simulink model "gm_combinedTxRx_ExternalMode"  (R2017b)
settings: Solver=FixedStepDiscrete  StartTime=0.0  StopTime=10.0  RelTol=1e-3
InitFcn:
  | modelSettings
undefined symbols (not defined in the file or in its folder): coeff, filt, j, RadioSampleRate, VibertiTracebackLength, xPreambleSeq
libraries: simulink x20, dsphdlfiltering x20, hdlsllib x10, hdlmdlgenlib x6, dspsigops x5, commseqgen3 x4, commdigbbndpm3 x3, commcrc2 x2, commcnvcod2 x2, commsource2 x1, dspstat3 x1, dspmlti4 x1
(part 4 of 5)

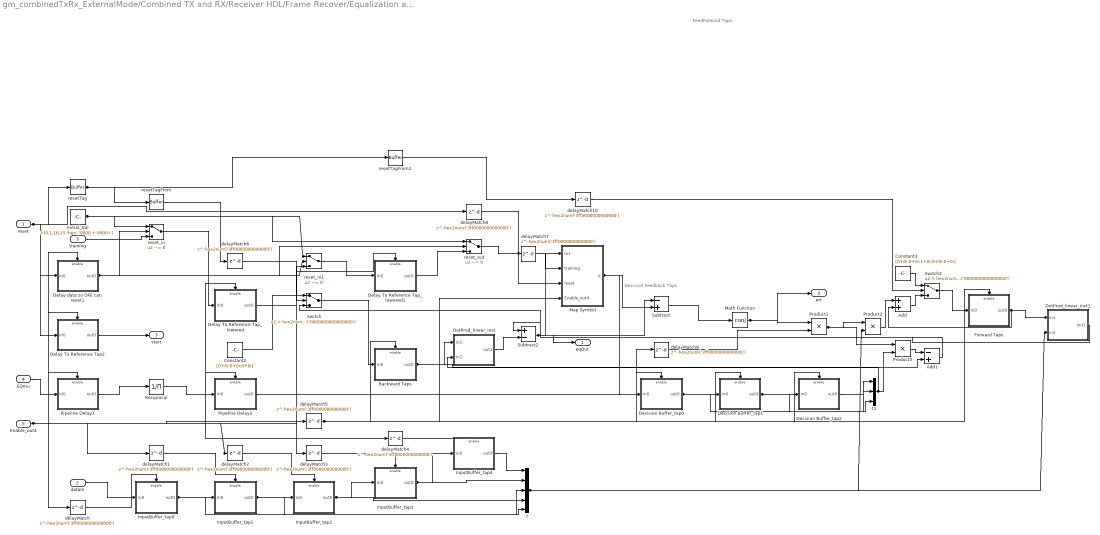
== system gm_combinedTxRx_ExternalMode/Combined TX and RX/Receiver HDL/Frame Recover/Equalization and Demodulation/DFE/DFE ==
  note: Decision Feedback Taps
  note: FeedForward Taps
  reset : Inport  SampleTime=1e-06
  dataIn : Inport  Port=2  OutDataTypeStr=fixdt(1,16,14)  SampleTime=1e-06
  training : Inport  Port=3  OutDataTypeStr=fixdt(1,16,15)  SampleTime=1e-06
  EQmu : Inport  Port=4  SampleTime=1e-06
  Enable_out4 : Inport  Port=5  OutDataTypeStr=boolean  SampleTime=1e-06
  Add : Sum  AccumDataTypeStr=fixdt(1, 25, 22)  OutDataTypeStr=fixdt(1, 16, 14)  SampleTime=1e-06
  Add1 : Sum  Inputs=-+  AccumDataTypeStr=fixdt(1, 23, 21)  OutDataTypeStr=fixdt(1, 16, 19)  SampleTime=1e-06
  Backward Taps : Subsystem
      settings: MinAlgLoopOccurrences=on
  Constant2 : Constant  Value=[0+0i;0+0i;0+0i]  OutDataTypeStr=fixdt(1, 16, 4)  SampleTime=-1
  Constant3 : Constant  Value=[0+0i;0+0i;1+0i;0+0i;0+0i]  OutDataTypeStr=fixdt(1, 16, 4)  SampleTime=-1
  Decision Buffer_tap0 : Subsystem
      settings: MinAlgLoopOccurrences=on
  Decision Buffer_tap1 : Subsystem
      settings: MinAlgLoopOccurrences=on
  Decision Buffer_tap2 : Subsystem
      settings: MinAlgLoopOccurrences=on
  Delay To Reference Tap2 : Subsystem
      settings: MinAlgLoopOccurrences=on
  Delay To Reference Tap_lowered : Subsystem
      settings: MinAlgLoopOccurrences=on
  Delay To Reference Tap_lowered1 : Subsystem
      settings: MinAlgLoopOccurrences=on
  Delay data so DFE can reset1 : Subsystem
      settings: MinAlgLoopOccurrences=on
  DotProd_linear_inst : Subsystem
  DotProd_linear_inst1 : Subsystem
  Forward Taps : Subsystem
      settings: MinAlgLoopOccurrences=on
  Initial_Val : Constant  Value=fi(0,1,16,15,'hex','0000 + 0000 i')  OutDataTypeStr=fixdt(1, 16, 15)  SampleTime=-1
  InputBuffer_tap0 : Subsystem
      settings: MinAlgLoopOccurrences=on
  InputBuffer_tap1 : Subsystem
      settings: MinAlgLoopOccurrences=on
  InputBuffer_tap2 : Subsystem
      settings: MinAlgLoopOccurrences=on
  InputBuffer_tap3 : Subsystem
      settings: MinAlgLoopOccurrences=on
  InputBuffer_tap4 : Subsystem
      settings: MinAlgLoopOccurrences=on
  Map Symbol : Subsystem
  Math Function : Math  Operator=conj  RndMeth=Zero  SaturateOnIntegerOverflow=on
  Pipeline Delay1 : Subsystem
      settings: MinAlgLoopOccurrences=on
  Pipeline Delay2 : Subsystem
      settings: MinAlgLoopOccurrences=on
  Product1 : Product  Inputs=**  OutDataTypeStr=fixdt(1, 16, 22)  SampleTime=1e-06
  Product2 : Product  Inputs=**  OutDataTypeStr=fixdt(1, 16, 22)  SampleTime=1e-06
  Product3 : Product  Inputs=**  OutDataTypeStr=fixdt(1, 16, 21)  SampleTime=1e-06
  Reciprocal : Product  Inputs=/  OutDataTypeStr=fixdt(0, 16, 22)  SampleTime=1e-06  SaturateOnIntegerOverflow=on  RndMeth=Zero
  Subtract : Sum  Inputs=-+  AccumDataTypeStr=fixdt(1, 18, 15)  OutDataTypeStr=fixdt(1, 16, 15)  SampleTime=1e-06
  Subtract2 : Sum  Inputs=+-  AccumDataTypeStr=fixdt(1, 21, 18)  OutDataTypeStr=fixdt(1, 16, 14)  SampleTime=1e-06
  Switch : Switch  Criteria=u2 > Threshold  Threshold=hex2num('0000000000000000')  OutDataTypeStr=fixdt(1, 16, 15)  SampleTime=1e-06
  Switch2 : Switch  Criteria=u2 > Threshold  Threshold=hex2num('0000000000000000')  OutDataTypeStr=fixdt(1, 16, 14)  SampleTime=1e-06
  delayMatch{,1..10} (11 alike) : Delay  DelayLength=hex2num('3ff0000000000000')  InitialCondition=0  InputProcessing=Inherited
  resetTag : hdlmdlgenlib/Buffer
      settings: SourceProductName=HDL Coder  SourceProductBaseCode=HD
  resetTagFrom : hdlmdlgenlib/Buffer
      settings: SourceProductName=HDL Coder  SourceProductBaseCode=HD
  resetTagFrom1 : hdlmdlgenlib/Buffer
      settings: SourceProductName=HDL Coder  SourceProductBaseCode=HD
  reset_in : Switch  Criteria=u2 ~= 0  Threshold=hex2num('0000000000000000')  OutDataTypeStr=fixdt(1, 16, 15)  SampleTime=1e-06
  reset_in1 : Switch  Criteria=u2 ~= 0  Threshold=hex2num('0000000000000000')  OutDataTypeStr=fixdt(1, 16, 15)  SampleTime=1e-06
  reset_out : Switch  Criteria=u2 ~= 0  Threshold=hex2num('0000000000000000')  OutDataTypeStr=fixdt(1, 16, 15)  SampleTime=1e-06
  t : Mux  Inputs=5
  t1 : Mux  Inputs=3
  eqOut : Outport  InitialOutput=0
  err : Outport  Port=2  InitialOutput=0
  start : Outport  Port=3  InitialOutput=0
  wires:
  delayMatch8/1 -> Map Symbol/3(reset)
  Constant2/1 -> Switch/1
  Constant3/1 -> Switch2/1
  delayMatch7/1 -> Map Symbol/2(training)
  Delay To Reference Tap2/1(out0) -> start/1
  Delay data so DFE can reset1/1(out0) -> reset_out/2, reset_in1/2, reset_in/2
  t/1 -> Product2/2, DotProd_linear_inst1/2(in2)
  Pipeline Delay1/1(out0) -> Reciprocal/1
  delayMatch9/1 -> Product1/2
  Reciprocal/1 -> Pipeline Delay2/1(in0)
  delayMatch6/1 -> Switch/2
  delayMatch10/1 -> Switch2/2
  resetTag/1 -> resetTagFrom1/1, resetTagFrom/1
  Initial_Val/1 -> reset_out/1, reset_in1/1, reset_in/1
  Delay To Reference Tap_lowered/1(out0) -> reset_in1/3
  reset_in/1 -> Delay To Reference Tap_lowered/1(in0)
  Delay To Reference Tap_lowered1/1(out0) -> reset_out/3
  reset_in1/1 -> Delay To Reference Tap_lowered1/1(in0)
  InputBuffer_tap0/1(out0) -> InputBuffer_tap1/1(in0), t/5
  InputBuffer_tap1/1(out0) -> InputBuffer_tap2/1(in0), t/4
  InputBuffer_tap2/1(out0) -> InputBuffer_tap3/1(in0), t/3
  InputBuffer_tap3/1(out0) -> InputBuffer_tap4/1(in0), t/2
  InputBuffer_tap4/1(out0) -> t/1
  delayMatch/1 -> InputBuffer_tap0/Enable
  reset/1 -> delayMatch8/1, Delay data so DFE can reset1/1(in0), Delay To Reference Tap2/1(in0), resetTag/1
  dataIn/1 -> InputBuffer_tap0/1(in0)
  training/1 -> reset_in/3
  EQmu/1 -> Pipeline Delay1/1(in0)
  Enable_out4/1 -> delayMatch5/1, delayMatch4/1, delayMatch3/1, delayMatch2/1, delayMatch1/1, delayMatch/1, Delay To Reference Tap_lowered1/Enable, Delay To Reference Tap_lowered/Enable, Pipeline Delay2/Enable, Pipeline Delay1/Enable, Delay data so DFE can reset1/Enable, Delay To Reference Tap2/Enable
  delayMatch1/1 -> InputBuffer_tap1/Enable
  delayMatch2/1 -> InputBuffer_tap2/Enable
  delayMatch3/1 -> InputBuffer_tap3/Enable
  delayMatch4/1 -> InputBuffer_tap4/Enable
  delayMatch5/1 -> Decision Buffer_tap2/Enable, Decision Buffer_tap1/Enable, Decision Buffer_tap0/Enable, Forward Taps/Enable, Backward Taps/Enable, Map Symbol/4(Enable_out4)
  resetTagFrom/1 -> delayMatch6/1
  reset_out/1 -> delayMatch7/1
  Pipeline Delay2/1(out0) -> delayMatch9/1
  resetTagFrom1/1 -> delayMatch10/1
  Decision Buffer_tap0/1(out0) -> Decision Buffer_tap1/1(in0), t1/3
  Decision Buffer_tap1/1(out0) -> Decision Buffer_tap2/1(in0), t1/2
  Decision Buffer_tap2/1(out0) -> t1/1
  t1/1 -> Product3/2, DotProd_linear_inst/2(in2)
  Product3/1 -> Add1/1
  Add1/1 -> Switch/3
  Switch/1 -> Backward Taps/1(in0)
  Backward Taps/1(out0) -> DotProd_linear_inst/1(in1), Add1/2
  DotProd_linear_inst/1(out1) -> Subtract2/2
  Map Symbol/1(d) -> Subtract/2, Decision Buffer_tap0/1(in0)
  Subtract/1 -> Math Function/1
  Product1/1 -> Product3/1, Product2/1
  Product2/1 -> Add/1
  Add/1 -> Switch2/3
  Switch2/1 -> Forward Taps/1(in0)
  Forward Taps/1(out0) -> DotProd_linear_inst1/1(in1), Add/2
  DotProd_linear_inst1/1(out1) -> Subtract2/1
  Math Function/1 -> Product1/1, err/1
  Subtract2/1 -> Subtract/1, Map Symbol/1(In1), eqOut/1

== system gm_combinedTxRx_ExternalMode/Combined TX and RX/Receiver HDL/Frame Recover/Equalization and Demodulation/DFE/Delay data so DFE can reset ==
  in0 : Inport  OutDataTypeStr=fixdt(1, 16, 14)  SampleTime=1e-06
      settings: SignalType=complex
  Enable_out4 : EnablePort  OutDataTypeStr=boolean
  Delay data so DFE can reset : Delay  DelayLength=hex2num('3ff0000000000000')  InitialCondition=0  InputProcessing=Inherited
  out0 : Outport  OutDataTypeStr=fixdt(1, 16, 14)  InitialOutput=0
      settings: SignalType=complex
  wires:
  Delay data so DFE can reset/1 -> out0/1
  in0/1 -> Delay data so DFE can reset/1

== system gm_combinedTxRx_ExternalMode/Combined TX and RX/Receiver HDL/Frame Recover/Equalization and Demodulation/DFE/Delay ref so DFE can reset ==
  in0 : Inport  OutDataTypeStr=fixdt(1, 16, 15)  SampleTime=1e-06
      settings: SignalType=complex
  Enable_out4 : EnablePort  OutDataTypeStr=boolean
  Delay ref so DFE can reset : Delay  DelayLength=hex2num('3ff0000000000000')  InitialCondition=0  InputProcessing=Inherited
  out0 : Outport  OutDataTypeStr=fixdt(1, 16, 15)  InitialOutput=0
      settings: SignalType=complex
  wires:
  Delay ref so DFE can reset/1 -> out0/1
  in0/1 -> Delay ref so DFE can reset/1

== system gm_combinedTxRx_ExternalMode/Combined TX and RX/Receiver HDL/Frame Recover/Equalization and Demodulation/DFE/PN Sequence Generator ==
  in0 : Inport  OutDataTypeStr=boolean  SampleTime=1e-06
  Enable_out4 : EnablePort  OutDataTypeStr=boolean
  PN Sequence Generator : commseqgen3/PN Sequence Generator  poly='z^5 + z^3 + z^1 + 1'  ini_sta=[1 1 1 0 0]  outBitMaskSource=Dialog parameter  shift=0  outVarSiz=off  maxOutSizeMode=Dialog parameter  maxOutSize=[10 1]  Ts=-1  sampPerFrame=1  reset=on  bitPackedOutputs=on  outDataType=Smallest unsigned integer  numPackedBits=2  bitPackDataSigned=off  bitPackedOutDType=Smallest integer
      settings: SourceProductName=Communications System Toolbox
  out0 : Outport  OutDataTypeStr=fixdt(0, 2, 0)  InitialOutput=0
  wires:
  PN Sequence Generator/1 -> out0/1
  in0/1 -> PN Sequence Generator/1

== system gm_combinedTxRx_ExternalMode/Combined TX and RX/Receiver HDL/Frame Recover/Equalization and Demodulation/DFE/Packeted To Unpacked ==
  In1 : Inport  SampleTime=1e-06
  Extract Bits : simulink/Logic and Bit Operations/Extract Bits  bitsToExtract=Range of bits  numBits=8  bitIdxRange=[1]  outScalingMode=Treat bit field as an integer
      settings: SourceProductName=Simulink
  Extract Bits1 : simulink/Logic and Bit Operations/Extract Bits  bitsToExtract=Range of bits  numBits=8  bitIdxRange=[0]  outScalingMode=Treat bit field as an integer
      settings: SourceProductName=Simulink
  Vector Concatenate : Concatenate
  Out1 : Outport  InitialOutput=0
  wires:
  Extract Bits/1 -> Vector Concatenate/1
  Extract Bits1/1 -> Vector Concatenate/2
  Vector Concatenate/1 -> Out1/1
  In1/1 -> Extract Bits1/1, Extract Bits/1

== system gm_combinedTxRx_ExternalMode/Combined TX and RX/Receiver HDL/Frame Recover/Equalization and Demodulation/DFE/QPSK Modulator Baseband ==
  in0 : Inport  OutDataTypeStr=fixdt(0, 1, 0)  PortDimensions=[2]  SampleTime=1e-06
  Enable_out4 : EnablePort  OutDataTypeStr=boolean
  QPSK Modulator Baseband : commdigbbndpm3/QPSK Modulator Baseband  InType=Bit  Enc=Binary  Ph=pi/4  outDtype=Fixed-point  outWordLen=16  outUDDataType=sfix(16)  outFracLenMode=User-defined  outFracLen=15  outDataTypeStr=fixdt(1,16,15)  outLastDataTypeStr=fixdt(1,16,15)
  out0 : Outport  OutDataTypeStr=fixdt(1, 16, 15)  InitialOutput=0
      settings: SignalType=complex
  wires:
  QPSK Modulator Baseband/1 -> out0/1
  in0/1 -> QPSK Modulator Baseband/1

== system gm_combinedTxRx_ExternalMode/Combined TX and RX/Receiver HDL/Frame Recover/Equalization and Demodulation/Header Controller/Header Controller ==
  headerStart : Inport  SampleTime=1e-06
  data : Inport  Port=2  PortDimensions=2  SampleTime=1e-06
  RxTxFixedPointLibrary_c15_Header_Controller : MATLAB Function  TreatAsAtomicUnit=on
  enableDownstream : Outport  InitialOutput=0
  packetLenBitsOut : Outport  Port=2  InitialOutput=0
  resetViterbi : Outport  Port=3  InitialOutput=0
  crcStart : Outport  Port=4  InitialOutput=0
  status : Outport  Port=5  InitialOutput=0
  s1 : Outport  Port=6  InitialOutput=0
  s2 : Outport  Port=7  InitialOutput=0
  wires:
  headerStart/1 -> RxTxFixedPointLibrary_c15_Header_Controller/1(headerStart)
  data/1 -> RxTxFixedPointLibrary_c15_Header_Controller/2(data)
  RxTxFixedPointLibrary_c15_Header_Controller/1(enableDownstream) -> enableDownstream/1
  RxTxFixedPointLibrary_c15_Header_Controller/2(packetLenBitsOut) -> packetLenBitsOut/1
  RxTxFixedPointLibrary_c15_Header_Controller/3(resetViterbi) -> resetViterbi/1
  RxTxFixedPointLibrary_c15_Header_Controller/4(crcStart) -> crcStart/1
  RxTxFixedPointLibrary_c15_Header_Controller/5(status) -> status/1
  RxTxFixedPointLibrary_c15_Header_Controller/6(s1) -> s1/1
  RxTxFixedPointLibrary_c15_Header_Controller/7(s2) -> s2/1

== system gm_combinedTxRx_ExternalMode/Combined TX and RX/Receiver HDL/Frame Recover/Frequency Recovery/Lock Detector/MATLAB Function ==
  u : Inport  SampleTime=1e-06
  RxTxFixedPointLibrary_c1_MATLAB_Function : MATLAB Function  TreatAsAtomicUnit=on
  y : Outport  InitialOutput=0
  wires:
  RxTxFixedPointLibrary_c1_MATLAB_Function/1(y) -> y/1
  u/1 -> RxTxFixedPointLibrary_c1_MATLAB_Function/1(u)

== system gm_combinedTxRx_ExternalMode/Combined TX and RX/Receiver HDL/Frame Recover/Frequency Recovery/Lock Detector/Pipeline Delay ==
  in0 : Inport  OutDataTypeStr=fixdt(1, 16, 10)  SampleTime=1e-06
  Enable_out4 : EnablePort  OutDataTypeStr=boolean
  Pipeline Delay : Delay  DelayLength=hex2num('3ff0000000000000')  InitialCondition=0  InputProcessing=Inherited
  out0 : Outport  OutDataTypeStr=fixdt(1, 16, 10)  InitialOutput=0
  wires:
  Pipeline Delay/1 -> out0/1
  in0/1 -> Pipeline Delay/1

== system gm_combinedTxRx_ExternalMode/Combined TX and RX/Receiver HDL/Frame Recover/Frequency Recovery/Lock Detector/Tapped Delay ==
  in0 : Inport  OutDataTypeStr=fixdt(0, 16, 10)  SampleTime=1e-06
  Enable_out4 : EnablePort  OutDataTypeStr=boolean
  Tapped Delay : simulink/Discrete/Tapped Delay  vinit=0  samptime=-1  NumDelays=hex2num('4059000000000000')  DelayOrder=Oldest  includeCurrent=off
  out0 : Outport  OutDataTypeStr=fixdt(0, 16, 10)  PortDimensions=[100]  InitialOutput=0
  wires:
  Tapped Delay/1 -> out0/1
  in0/1 -> Tapped Delay/1

== system gm_combinedTxRx_ExternalMode/Combined TX and RX/Receiver HDL/Frame Recover/Frequency Recovery/Loop Filter Configurable/Delay ==
  in0 : Inport  OutDataTypeStr=fixdt(1, 16, 10)  SampleTime=1e-06
  Enable_out4 : EnablePort  OutDataTypeStr=boolean
  Delay : Delay  DelayLength=hex2num('3ff0000000000000')  InitialCondition=0  InputProcessing=Inherited
  out0 : Outport  OutDataTypeStr=fixdt(1, 16, 10)  InitialOutput=0
  wires:
  Delay/1 -> out0/1
  in0/1 -> Delay/1

== system gm_combinedTxRx_ExternalMode/Combined TX and RX/Receiver HDL/Frame Recover/Frequency Recovery/Loop Filter Configurable/Delay3 ==
  in0 : Inport  OutDataTypeStr=fixdt(1, 16, 10)  SampleTime=1e-06
  Enable_out4 : EnablePort  OutDataTypeStr=boolean
  Delay3 : Delay  DelayLength=hex2num('3ff0000000000000')  InitialCondition=0  InputProcessing=Inherited
  out0 : Outport  OutDataTypeStr=fixdt(1, 16, 10)  InitialOutput=0
  wires:
  Delay3/1 -> out0/1
  in0/1 -> Delay3/1

== system gm_combinedTxRx_ExternalMode/Combined TX and RX/Receiver HDL/Frame Recover/Frequency Recovery/Loop Filter Configurable/Delay4 ==
  in0 : Inport  OutDataTypeStr=fixdt(1, 16, 10)  SampleTime=1e-06
  Enable_out4 : EnablePort  OutDataTypeStr=boolean
  Delay4 : Delay  DelayLength=hex2num('3ff0000000000000')  InitialCondition=0  InputProcessing=Inherited
  out0 : Outport  OutDataTypeStr=fixdt(1, 16, 10)  InitialOutput=0
  wires:
  Delay4/1 -> out0/1
  in0/1 -> Delay4/1

== system gm_combinedTxRx_ExternalMode/Combined TX and RX/Receiver HDL/Frame Recover/Gardner Timing Recovery/Gardner TED Blocks/Imag Error ==
  data : Inport  SampleTime=1e-06
  strobe sum : Inport  Port=2  SampleTime=1e-06
  Enable_out2 : Inport  Port=3  OutDataTypeStr=boolean  SampleTime=1e-06
  Delay : Subsystem
      settings: MinAlgLoopOccurrences=on
  Product1 : Product  Inputs=**  OutDataTypeStr=fixdt(1, 32, 20)  SampleTime=1e-06
  Sub : Sum  Inputs=+-  AccumDataTypeStr=fixdt(1, 16, 10)  OutDataTypeStr=fixdt(1, 16, 10)  SampleTime=1e-06
  TED Buffer Update1 : Subsystem
  Out1 : Outport  InitialOutput=0
  wires:
  data/1 -> Sub/2, Delay/1(in0)
  strobe sum/1 -> TED Buffer Update1/2(strobe sum)
  Delay/1(out0) -> TED Buffer Update1/1(new data)
  Product1/1 -> Out1/1
  Sub/1 -> Product1/2
  TED Buffer Update1/1(Middle Indx) -> Product1/1
  TED Buffer Update1/2(oldest) -> Sub/1
  Enable_out2/1 -> Delay/Enable, TED Buffer Update1/3(Enable_out2)

== system gm_combinedTxRx_ExternalMode/Combined TX and RX/Receiver HDL/Frame Recover/Gardner Timing Recovery/Gardner TED Blocks/Real Error ==
  data : Inport  SampleTime=1e-06
  strobe sum : Inport  Port=2  SampleTime=1e-06
  Enable_out2 : Inport  Port=3  OutDataTypeStr=boolean  SampleTime=1e-06
  Delay : Subsystem
      settings: MinAlgLoopOccurrences=on
  Product1 : Product  Inputs=**  OutDataTypeStr=fixdt(1, 16, 12)  SampleTime=1e-06
  Sub : Sum  Inputs=+-  AccumDataTypeStr=fixdt(1, 16, 10)  OutDataTypeStr=fixdt(1, 16, 10)  SampleTime=1e-06
  TED Buffer Update1 : Subsystem
  Out1 : Outport  InitialOutput=0
  wires:
  data/1 -> Sub/2, Delay/1(in0)
  strobe sum/1 -> TED Buffer Update1/2(strobe sum)
  Delay/1(out0) -> TED Buffer Update1/1(new data)
  Product1/1 -> Out1/1
  Sub/1 -> Product1/2
  TED Buffer Update1/1(Middle Indx) -> Product1/1
  TED Buffer Update1/2(oldest) -> Sub/1
  Enable_out2/1 -> Delay/Enable, TED Buffer Update1/3(Enable_out2)

== system gm_combinedTxRx_ExternalMode/Combined TX and RX/Receiver HDL/Frame Recover/Gardner Timing Recovery/Gardner TED Blocks/Strobe Buffer1_tap1 ==
  in0 : Inport  OutDataTypeStr=boolean  SampleTime=1e-06
  Enable_out2 : EnablePort  OutDataTypeStr=boolean
  Strobe Buffer1_tap1 : Delay  DelayLength=hex2num('3ff0000000000000')  InputProcessing=Inherited
  out0 : Outport  OutDataTypeStr=boolean  InitialOutput=0
  wires:
  Strobe Buffer1_tap1/1 -> out0/1
  in0/1 -> Strobe Buffer1_tap1/1

== system gm_combinedTxRx_ExternalMode/Combined TX and RX/Receiver HDL/Frame Recover/Gardner Timing Recovery/Gardner TED Blocks/Strobe Buffer1_tap2 ==
  in0 : Inport  OutDataTypeStr=boolean  SampleTime=1e-06
  Enable_out2 : EnablePort  OutDataTypeStr=boolean
  Strobe Buffer1_tap2 : Delay  DelayLength=hex2num('3ff0000000000000')  InputProcessing=Inherited
  out0 : Outport  OutDataTypeStr=boolean  InitialOutput=0
  wires:
  Strobe Buffer1_tap2/1 -> out0/1
  in0/1 -> Strobe Buffer1_tap2/1

== system gm_combinedTxRx_ExternalMode/Combined TX and RX/Receiver HDL/Frame Recover/Gardner Timing Recovery/Gardner TED Blocks/Strobe Buffer1_tap3 ==
  in0 : Inport  OutDataTypeStr=boolean  SampleTime=1e-06
  Enable_out2 : EnablePort  OutDataTypeStr=boolean
  Strobe Buffer1_tap3 : Delay  DelayLength=hex2num('3ff0000000000000')  InputProcessing=Inherited
  out0 : Outport  OutDataTypeStr=boolean  InitialOutput=0
  wires:
  Strobe Buffer1_tap3/1 -> out0/1
  in0/1 -> Strobe Buffer1_tap3/1

== system gm_combinedTxRx_ExternalMode/Combined TX and RX/Receiver HDL/Frame Recover/Gardner Timing Recovery/InterpControl_Blocks1/Calculate New mu ==
  note: Good at fixd(0,16,12)
  W : Inport  SampleTime=1e-06
  NCOCounter : Inport  Port=2  SampleTime=1e-06
  Math Reciprocal : Math  Operator=reciprocal  OutDataTypeStr=fixdt(1,16,12)  RndMeth=Zero  SaturateOnIntegerOverflow=on
  Product : Product  OutDataTypeStr=fixdt(0,15,14)
  mu : Outport  InitialOutput=0
  wires:
  W/1 -> Math Reciprocal/1
  NCOCounter/1 -> Product/2
  Math Reciprocal/1 -> Product/1
  Product/1 -> mu/1

== system gm_combinedTxRx_ExternalMode/Combined TX and RX/Receiver HDL/Frame Recover/Gardner Timing Recovery/InterpControl_Blocks1/Mod 1 ==
  In1 : Inport  SampleTime=1e-06
  Add : Sum
  Compare To Constant : simulink/Logic and Bit Operations/Compare To Constant  relop=<  const=1  OutDataTypeStr=boolean
  Compare To Constant1 : simulink/Logic and Bit Operations/Compare To Constant  relop=>=  const=0  OutDataTypeStr=boolean
  Constant : Constant  OutDataTypeStr=fixdt(0,1,0)  SampleTime=-1
  Constant1 : Constant  OutDataTypeStr=fixdt(0,1,0)  SampleTime=-1
  Logical Operator : Logic  AllPortsSameDT=off  OutDataTypeStr=boolean
  Subtract : Sum  Inputs=+-
  Switch : Switch  Criteria=u2 > Threshold
  Switch1 : Switch
  Out1 : Outport  InitialOutput=0
  wires:
  In1/1 -> Switch1/2, Switch/1, Subtract/1, Compare To Constant1/1, Compare To Constant/1, Add/1
  Add/1 -> Switch1/3
  Compare To Constant/1 -> Logical Operator/2
  Compare To Constant1/1 -> Logical Operator/1
  Constant/1 -> Subtract/2
  Constant1/1 -> Add/2
  Logical Operator/1 -> Switch/2
  Subtract/1 -> Switch1/1
  Switch/1 -> Out1/1
  Switch1/1 -> Switch/3

== system gm_combinedTxRx_ExternalMode/Combined TX and RX/Receiver HDL/Frame Recover/Gardner Timing Recovery/InterpControl_Blocks1/NCOCounter State ==
  in0 : Inport  OutDataTypeStr=fixdt(0, 16, 16)  SampleTime=1e-06
  Enable_out2 : EnablePort  OutDataTypeStr=boolean
  NCOCounter State : Delay  DelayLength=hex2num('3ff0000000000000')  InitialCondition=0  InputProcessing=Inherited
  out0 : Outport  OutDataTypeStr=fixdt(0, 16, 16)  InitialOutput=0
  wires:
  NCOCounter State/1 -> out0/1
  in0/1 -> NCOCounter State/1

== system gm_combinedTxRx_ExternalMode/Combined TX and RX/Receiver HDL/Frame Recover/Gardner Timing Recovery/InterpControl_Blocks1/saved mu ==
  in0 : Inport  OutDataTypeStr=fixdt(0, 15, 14)  SampleTime=1e-06
  Enable_out2 : EnablePort  OutDataTypeStr=boolean
  saved mu : Delay  DelayLength=hex2num('3ff0000000000000')  InitialCondition=0  InputProcessing=Inherited
  out0 : Outport  OutDataTypeStr=fixdt(0, 15, 14)  InitialOutput=0
  wires:
  saved mu/1 -> out0/1
  in0/1 -> saved mu/1

== system gm_combinedTxRx_ExternalMode/Combined TX and RX/Receiver HDL/Frame Recover/Gardner Timing Recovery/Interpolator/Delay ==
  in0 : Inport  OutDataTypeStr=fixdt(1, 16, 14)  SampleTime=1e-06
      settings: SignalType=complex
  Enable_out2 : EnablePort  OutDataTypeStr=boolean
  Delay : Delay  DelayLength=hex2num('3ff0000000000000')  InitialCondition=0  InputProcessing=Inherited
  out0 : Outport  OutDataTypeStr=fixdt(1, 16, 14)  InitialOutput=0
      settings: SignalType=complex
  wires:
  Delay/1 -> out0/1
  in0/1 -> Delay/1

== system gm_combinedTxRx_ExternalMode/Combined TX and RX/Receiver HDL/Frame Recover/Gardner Timing Recovery/Interpolator/Delay1 ==
  in0 : Inport  OutDataTypeStr=fixdt(1, 16, 14)  SampleTime=1e-06
      settings: SignalType=complex
  Enable_out2 : EnablePort  OutDataTypeStr=boolean
  Delay1 : Delay  DelayLength=hex2num('3ff0000000000000')  InitialCondition=0  InputProcessing=Inherited
  out0 : Outport  OutDataTypeStr=fixdt(1, 16, 14)  InitialOutput=0
      settings: SignalType=complex
  wires:
  Delay1/1 -> out0/1
  in0/1 -> Delay1/1

== system gm_combinedTxRx_ExternalMode/Combined TX and RX/Receiver HDL/Frame Recover/Gardner Timing Recovery/Interpolator/Delay2 ==
  in0 : Inport  OutDataTypeStr=fixdt(1, 16, 14)  SampleTime=1e-06
      settings: SignalType=complex
  Enable_out2 : EnablePort  OutDataTypeStr=boolean
  Delay2 : Delay  DelayLength=hex2num('3ff0000000000000')  InitialCondition=0  InputProcessing=Inherited
  out0 : Outport  OutDataTypeStr=fixdt(1, 16, 14)  InitialOutput=0
      settings: SignalType=complex
  wires:
  Delay2/1 -> out0/1
  in0/1 -> Delay2/1

== system gm_combinedTxRx_ExternalMode/Combined TX and RX/Receiver HDL/Frame Recover/Gardner Timing Recovery/Interpolator/Delay3 ==
  in0 : Inport  OutDataTypeStr=fixdt(1, 16, 13)  SampleTime=1e-06
      settings: SignalType=complex
  Enable_out2 : EnablePort  OutDataTypeStr=boolean
  Delay3 : Delay  DelayLength=hex2num('3ff0000000000000')  InitialCondition=0  InputProcessing=Inherited
  out0 : Outport  OutDataTypeStr=fixdt(1, 16, 13)  InitialOutput=0
      settings: SignalType=complex
  wires:
  Delay3/1 -> out0/1
  in0/1 -> Delay3/1

== system gm_combinedTxRx_ExternalMode/Combined TX and RX/Receiver HDL/Frame Recover/Gardner Timing Recovery/Interpolator/Delay4 ==
  in0 : Inport  OutDataTypeStr=fixdt(1, 16, 13)  SampleTime=1e-06
      settings: SignalType=complex
  Enable_out2 : EnablePort  OutDataTypeStr=boolean
  Delay4 : Delay  DelayLength=hex2num('3ff0000000000000')  InitialCondition=0  InputProcessing=Inherited
  out0 : Outport  OutDataTypeStr=fixdt(1, 16, 13)  InitialOutput=0
      settings: SignalType=complex
  wires:
  Delay4/1 -> out0/1
  in0/1 -> Delay4/1

== system gm_combinedTxRx_ExternalMode/Combined TX and RX/Receiver HDL/Frame Recover/Gardner Timing Recovery/Interpolator/PLD ==
  in0 : Inport  OutDataTypeStr=fixdt(1, 20, 14)  SampleTime=1e-06
      settings: SignalType=complex
  Enable_out2 : EnablePort  OutDataTypeStr=boolean
  PLD : Delay  DelayLength=hex2num('3ff0000000000000')  InitialCondition=0  InputProcessing=Inherited
  out0 : Outport  OutDataTypeStr=fixdt(1, 20, 14)  InitialOutput=0
      settings: SignalType=complex
  wires:
  PLD/1 -> out0/1
  in0/1 -> PLD/1

== system gm_combinedTxRx_ExternalMode/Combined TX and RX/Receiver HDL/Frame Recover/Gardner Timing Recovery/Interpolator/PLD1 ==
  in0 : Inport  OutDataTypeStr=fixdt(1, 18, 14)  SampleTime=1e-06
      settings: SignalType=complex
  Enable_out2 : EnablePort  OutDataTypeStr=boolean
  PLD1 : Delay  DelayLength=hex2num('3ff0000000000000')  InitialCondition=0  InputProcessing=Inherited
  out0 : Outport  OutDataTypeStr=fixdt(1, 18, 14)  InitialOutput=0
      settings: SignalType=complex
  wires:
  PLD1/1 -> out0/1
  in0/1 -> PLD1/1

== system gm_combinedTxRx_ExternalMode/Combined TX and RX/Receiver HDL/Frame Recover/Gardner Timing Recovery/Interpolator/PLD2 ==
  in0 : Inport  OutDataTypeStr=fixdt(0, 15, 14)  SampleTime=1e-06
  Enable_out2 : EnablePort  OutDataTypeStr=boolean
  PLD2 : Delay  DelayLength=hex2num('3ff0000000000000')  InitialCondition=0  InputProcessing=Inherited
  out0 : Outport  OutDataTypeStr=fixdt(0, 15, 14)  InitialOutput=0
  wires:
  PLD2/1 -> out0/1
  in0/1 -> PLD2/1

== system gm_combinedTxRx_ExternalMode/Combined TX and RX/Receiver HDL/Frame Recover/Gardner Timing Recovery/Interpolator/PLD3 ==
  in0 : Inport  OutDataTypeStr=fixdt(1, 16, 13)  SampleTime=1e-06
      settings: SignalType=complex
  Enable_out2 : EnablePort  OutDataTypeStr=boolean
  PLD3 : Delay  DelayLength=hex2num('3ff0000000000000')  InitialCondition=0  InputProcessing=Inherited
  out0 : Outport  OutDataTypeStr=fixdt(1, 16, 13)  InitialOutput=0
      settings: SignalType=complex
  wires:
  PLD3/1 -> out0/1
  in0/1 -> PLD3/1

== system gm_combinedTxRx_ExternalMode/Combined TX and RX/Receiver HDL/Frame Recover/Gardner Timing Recovery/Interpolator/PLD4 ==
  in0 : Inport  OutDataTypeStr=fixdt(1, 16, 13)  SampleTime=1e-06
      settings: SignalType=complex
  Enable_out2 : EnablePort  OutDataTypeStr=boolean
  PLD4 : Delay  DelayLength=hex2num('3ff0000000000000')  InitialCondition=0  InputProcessing=Inherited
  out0 : Outport  OutDataTypeStr=fixdt(1, 16, 13)  InitialOutput=0
      settings: SignalType=complex
  wires:
  PLD4/1 -> out0/1
  in0/1 -> PLD4/1

== system gm_combinedTxRx_ExternalMode/Combined TX and RX/Receiver HDL/Frame Recover/Gardner Timing Recovery/Interpolator/PLD5 ==
  in0 : Inport  OutDataTypeStr=fixdt(1, 21, 14)  SampleTime=1e-06
      settings: SignalType=complex
  Enable_out2 : EnablePort  OutDataTypeStr=boolean
  PLD5 : Delay  DelayLength=hex2num('3ff0000000000000')  InitialCondition=0  InputProcessing=Inherited
  out0 : Outport  OutDataTypeStr=fixdt(1, 21, 14)  InitialOutput=0
      settings: SignalType=complex
  wires:
  PLD5/1 -> out0/1
  in0/1 -> PLD5/1

== system gm_combinedTxRx_ExternalMode/Combined TX and RX/Receiver HDL/Frame Recover/Gardner Timing Recovery/Interpolator/PLD6 ==
  in0 : Inport  OutDataTypeStr=fixdt(0, 15, 14)  SampleTime=1e-06
  Enable_out2 : EnablePort  OutDataTypeStr=boolean
  PLD6 : Delay  DelayLength=hex2num('3ff0000000000000')  InitialCondition=0  InputProcessing=Inherited
  out0 : Outport  OutDataTypeStr=fixdt(0, 15, 14)  InitialOutput=0
  wires:
  PLD6/1 -> out0/1
  in0/1 -> PLD6/1

== system gm_combinedTxRx_ExternalMode/Combined TX and RX/Receiver HDL/Frame Recover/Gardner Timing Recovery/Interpolator/PLD7 ==
  in0 : Inport  OutDataTypeStr=fixdt(1, 16, 10)  SampleTime=1e-06
      settings: SignalType=complex
  Enable_out2 : EnablePort  OutDataTypeStr=boolean
  PLD7 : Delay  DelayLength=hex2num('4000000000000000')  InitialCondition=0  InputProcessing=Inherited
  out0 : Outport  OutDataTypeStr=fixdt(1, 16, 10)  InitialOutput=0
      settings: SignalType=complex
  wires:
  PLD7/1 -> out0/1
  in0/1 -> PLD7/1

== system gm_combinedTxRx_ExternalMode/Combined TX and RX/Receiver HDL/Frame Recover/Gardner Timing Recovery/LoopFilter1/Delay1 ==
  in0 : Inport  OutDataTypeStr=fixdt(1, 16, 24)  SampleTime=1e-06
  Enable_out2 : EnablePort  OutDataTypeStr=boolean
  Delay1 : Delay  DelayLength=hex2num('3ff0000000000000')  InitialCondition=0  InputProcessing=Inherited
  out0 : Outport  OutDataTypeStr=fixdt(1, 16, 24)  InitialOutput=0
  wires:
  Delay1/1 -> out0/1
  in0/1 -> Delay1/1

== system gm_combinedTxRx_ExternalMode/Combined TX and RX/Receiver HDL/Frame Recover/Gardner Timing Recovery/LoopFilter1/Delay2 ==
  in0 : Inport  OutDataTypeStr=fixdt(1, 16, 15)  SampleTime=1e-06
  Enable_out2 : EnablePort  OutDataTypeStr=boolean
  Delay2 : Delay  DelayLength=hex2num('3ff0000000000000')  InitialCondition=0  InputProcessing=Inherited
  out0 : Outport  OutDataTypeStr=fixdt(1, 16, 15)  InitialOutput=0
  wires:
  Delay2/1 -> out0/1
  in0/1 -> Delay2/1

== system gm_combinedTxRx_ExternalMode/Combined TX and RX/Receiver HDL/Frame Recover/Gardner Timing Recovery/TED Lock Detector/MATLAB Function ==
  u : Inport  SampleTime=1e-06
  RxTxFixedPointLibrary_c5_MATLAB_Function : MATLAB Function  TreatAsAtomicUnit=on
  y : Outport  InitialOutput=0
  wires:
  RxTxFixedPointLibrary_c5_MATLAB_Function/1(y) -> y/1
  u/1 -> RxTxFixedPointLibrary_c5_MATLAB_Function/1(u)

== system gm_combinedTxRx_ExternalMode/Combined TX and RX/Receiver HDL/Frame Recover/Gardner Timing Recovery/TED Lock Detector/Pipeline Delay ==
  in0 : Inport  OutDataTypeStr=fixdt(1, 16, 15)  SampleTime=1e-06
  Enable_out2 : EnablePort  OutDataTypeStr=boolean
  Pipeline Delay : Delay  DelayLength=hex2num('3ff0000000000000')  InitialCondition=0  InputProcessing=Inherited
  out0 : Outport  OutDataTypeStr=fixdt(1, 16, 15)  InitialOutput=0
  wires:
  Pipeline Delay/1 -> out0/1
  in0/1 -> Pipeline Delay/1

== system gm_combinedTxRx_ExternalMode/Combined TX and RX/Receiver HDL/Frame Recover/Gardner Timing Recovery/TED Lock Detector/Tapped Delay ==
  in0 : Inport  OutDataTypeStr=fixdt(0, 16, 15)  SampleTime=1e-06
  Enable_out2 : EnablePort  OutDataTypeStr=boolean
  Tapped Delay : simulink/Discrete/Tapped Delay  vinit=0  samptime=-1  NumDelays=hex2num('4059000000000000')  DelayOrder=Oldest  includeCurrent=off
  out0 : Outport  OutDataTypeStr=fixdt(0, 16, 15)  PortDimensions=[100]  InitialOutput=0
  wires:
  Tapped Delay/1 -> out0/1
  in0/1 -> Tapped Delay/1

== system gm_combinedTxRx_ExternalMode/Combined TX and RX/Transmitter HDL/Packet Generation/Payload/HDL Scrambler 2 bits/Buffer Manage ==
  bit1 : Inport  SampleTime=4e-06
  bit2 : Inport  Port=2  SampleTime=4e-06
  reset : Inport  Port=3  SampleTime=4e-06
  RxTxFixedPointLibrary_c20_Buffer_Manage : MATLAB Function  TreatAsAtomicUnit=on
  outBuffer : Outport
  wires:
  bit1/1 -> RxTxFixedPointLibrary_c20_Buffer_Manage/1(bit1)
  bit2/1 -> RxTxFixedPointLibrary_c20_Buffer_Manage/2(bit2)
  reset/1 -> RxTxFixedPointLibrary_c20_Buffer_Manage/3(reset)
  RxTxFixedPointLibrary_c20_Buffer_Manage/1(outBuffer) -> outBuffer/1

== system gm_combinedTxRx_ExternalMode/Combined TX and RX/Transmitter HDL/Packet Generation/Payload/Subsystem/MATLAB Function3 ==
  start : Inport  SampleTime=4e-06
  done : Inport  Port=2  SampleTime=4e-06
  RxTxFixedPointLibrary_c9_MATLAB_Function3 : MATLAB Function  TreatAsAtomicUnit=on
  enable : Outport
  wires:
  start/1 -> RxTxFixedPointLibrary_c9_MATLAB_Function3/1(start)
  done/1 -> RxTxFixedPointLibrary_c9_MATLAB_Function3/2(done)
  RxTxFixedPointLibrary_c9_MATLAB_Function3/1(enable) -> enable/1

== system gm_combinedTxRx_ExternalMode/Combined TX and RX/Receiver HDL/Frame Recover/Equalization and Demodulation/2 Bit Descrambler/MATLAB Function/MATLAB Function ==
  bits : Inport  PortDimensions=2  SampleTime=1e-06
  reset : Inport  Port=2  SampleTime=1e-06
  RxTxFixedPointLibrary_c10_MATLAB_Function : MATLAB Function  TreatAsAtomicUnit=on
  bufferA : Outport  InitialOutput=0
  bufferB : Outport  Port=2  InitialOutput=0
  wires:
  bits/1 -> RxTxFixedPointLibrary_c10_MATLAB_Function/1(bits)
  reset/1 -> RxTxFixedPointLibrary_c10_MATLAB_Function/2(reset)
  RxTxFixedPointLibrary_c10_MATLAB_Function/1(bufferA) -> bufferA/1
  RxTxFixedPointLibrary_c10_MATLAB_Function/2(bufferB) -> bufferB/1

== system gm_combinedTxRx_ExternalMode/Combined TX and RX/Receiver HDL/Frame Recover/Equalization and Demodulation/DFE/DFE/Backward Taps ==
  in0 : Inport  OutDataTypeStr=fixdt(1, 16, 15)  PortDimensions=[3]  SampleTime=1e-06
      settings: SignalType=complex
  Enable_out4 : EnablePort  OutDataTypeStr=boolean
  Backward Taps : UnitDelay  InitialCondition="[0  0  0]"  SampleTime=1e-06
  out0 : Outport  OutDataTypeStr=fixdt(1, 16, 15)  PortDimensions=[3]  InitialOutput=0
      settings: SignalType=complex
  wires:
  Backward Taps/1 -> out0/1
  in0/1 -> Backward Taps/1

== system gm_combinedTxRx_ExternalMode/Combined TX and RX/Receiver HDL/Frame Recover/Equalization and Demodulation/DFE/DFE/Decision Buffer_tap0 ==
  in0 : Inport  OutDataTypeStr=fixdt(1, 16, 15)  SampleTime=1e-06
      settings: SignalType=complex
  Enable_out4 : EnablePort  OutDataTypeStr=boolean
  Decision Buffer_tap0 : Delay  DelayLength=hex2num('3ff0000000000000')  InputProcessing=Inherited
  out0 : Outport  OutDataTypeStr=fixdt(1, 16, 15)  InitialOutput=0
      settings: SignalType=complex
  wires:
  Decision Buffer_tap0/1 -> out0/1
  in0/1 -> Decision Buffer_tap0/1

== system gm_combinedTxRx_ExternalMode/Combined TX and RX/Receiver HDL/Frame Recover/Equalization and Demodulation/DFE/DFE/Decision Buffer_tap1 ==
  in0 : Inport  OutDataTypeStr=fixdt(1, 16, 15)  SampleTime=1e-06
      settings: SignalType=complex
  Enable_out4 : EnablePort  OutDataTypeStr=boolean
  Decision Buffer_tap1 : Delay  DelayLength=hex2num('3ff0000000000000')  InputProcessing=Inherited
  out0 : Outport  OutDataTypeStr=fixdt(1, 16, 15)  InitialOutput=0
      settings: SignalType=complex
  wires:
  Decision Buffer_tap1/1 -> out0/1
  in0/1 -> Decision Buffer_tap1/1

== system gm_combinedTxRx_ExternalMode/Combined TX and RX/Receiver HDL/Frame Recover/Equalization and Demodulation/DFE/DFE/Decision Buffer_tap2 ==
  in0 : Inport  OutDataTypeStr=fixdt(1, 16, 15)  SampleTime=1e-06
      settings: SignalType=complex
  Enable_out4 : EnablePort  OutDataTypeStr=boolean
  Decision Buffer_tap2 : Delay  DelayLength=hex2num('3ff0000000000000')  InputProcessing=Inherited
  out0 : Outport  OutDataTypeStr=fixdt(1, 16, 15)  InitialOutput=0
      settings: SignalType=complex
  wires:
  Decision Buffer_tap2/1 -> out0/1
  in0/1 -> Decision Buffer_tap2/1

== system gm_combinedTxRx_ExternalMode/Combined TX and RX/Receiver HDL/Frame Recover/Equalization and Demodulation/DFE/DFE/Delay To Reference Tap2 ==
  in0 : Inport  OutDataTypeStr=boolean  SampleTime=1e-06
  Enable_out4 : EnablePort  OutDataTypeStr=boolean
  Delay To Reference Tap2 : Delay  DelayLength=hex2num('4008000000000000')  InitialCondition=0  InputProcessing=Inherited
  out0 : Outport  OutDataTypeStr=boolean  InitialOutput=0
  wires:
  Delay To Reference Tap2/1 -> out0/1
  in0/1 -> Delay To Reference Tap2/1

== system gm_combinedTxRx_ExternalMode/Combined TX and RX/Receiver HDL/Frame Recover/Equalization and Demodulation/DFE/DFE/Delay To Reference Tap_lowered ==
  in0 : Inport  OutDataTypeStr=fixdt(1, 16, 15)  SampleTime=1e-06
      settings: SignalType=complex
  Enable_out4 : EnablePort  OutDataTypeStr=boolean
  Delay To Reference Tap_lowered : Delay  DelayLength=hex2num('3ff0000000000000')  InitialCondition=0  InputProcessing=Inherited
  out0 : Outport  OutDataTypeStr=fixdt(1, 16, 15)  InitialOutput=0
      settings: SignalType=complex
  wires:
  Delay To Reference Tap_lowered/1 -> out0/1
  in0/1 -> Delay To Reference Tap_lowered/1

== system gm_combinedTxRx_ExternalMode/Combined TX and RX/Receiver HDL/Frame Recover/Equalization and Demodulation/DFE/DFE/Delay To Reference Tap_lowered1 ==
  in0 : Inport  OutDataTypeStr=fixdt(1, 16, 15)  SampleTime=1e-06
      settings: SignalType=complex
  Enable_out4 : EnablePort  OutDataTypeStr=boolean
  Delay To Reference Tap_lowered : Delay  DelayLength=hex2num('3ff0000000000000')  InitialCondition=0  InputProcessing=Inherited
  out0 : Outport  OutDataTypeStr=fixdt(1, 16, 15)  InitialOutput=0
      settings: SignalType=complex
  wires:
  Delay To Reference Tap_lowered/1 -> out0/1
  in0/1 -> Delay To Reference Tap_lowered/1

== system gm_combinedTxRx_ExternalMode/Combined TX and RX/Receiver HDL/Frame Recover/Equalization and Demodulation/DFE/DFE/Delay data so DFE can reset1 ==
  in0 : Inport  OutDataTypeStr=boolean  SampleTime=1e-06
  Enable_out4 : EnablePort  OutDataTypeStr=boolean
  Delay data so DFE can reset1 : Delay  DelayLength=hex2num('3ff0000000000000')  InitialCondition=0  InputProcessing=Inherited
  out0 : Outport  OutDataTypeStr=boolean  InitialOutput=0
  wires:
  Delay data so DFE can reset1/1 -> out0/1
  in0/1 -> Delay data so DFE can reset1/1

== system gm_combinedTxRx_ExternalMode/Combined TX and RX/Receiver HDL/Frame Recover/Equalization and Demodulation/DFE/DFE/DotProd_linear_inst ==
  in1 : Inport  OutDataTypeStr=fixdt(1, 16, 15)  PortDimensions=[3]  SampleTime=1e-06
      settings: SignalType=complex
  in2 : Inport  Port=2  OutDataTypeStr=fixdt(1, 16, 15)  PortDimensions=[3]  SampleTime=1e-06
      settings: SignalType=complex
  Dot_Product1 : Math  Operator=conj  SaturateOnIntegerOverflow=on
  Dot_Product11 : Sum  AccumDataTypeStr=fixdt(1, 16, 18)  OutDataTypeStr=fixdt(1, 16, 18)  SampleTime=1e-06  SaturateOnIntegerOverflow=on
  Dot_Product12 : Sum  AccumDataTypeStr=fixdt(1, 16, 18)  OutDataTypeStr=fixdt(1, 16, 18)  SampleTime=1e-06  SaturateOnIntegerOverflow=on
  mul_Dot_Product1_dotp_0 : Product  Inputs=**  OutDataTypeStr=fixdt(1, 16, 18)  SampleTime=1e-06  SaturateOnIntegerOverflow=on
  mul_Dot_Product1_dotp_1 : Product  Inputs=**  OutDataTypeStr=fixdt(1, 16, 18)  SampleTime=1e-06  SaturateOnIntegerOverflow=on
  mul_Dot_Product1_dotp_2 : Product  Inputs=**  OutDataTypeStr=fixdt(1, 16, 18)  SampleTime=1e-06  SaturateOnIntegerOverflow=on
  t : Demux  Outputs=3
  t1 : Demux  Outputs=3
  out1 : Outport  OutDataTypeStr=fixdt(1, 16, 18)
      settings: SignalType=complex
  wires:
  in1/1 -> Dot_Product1/1
  in2/1 -> t1/1
  Dot_Product12/1 -> out1/1
  Dot_Product1/1 -> t/1
  t/1 -> mul_Dot_Product1_dotp_0/1
  t/2 -> mul_Dot_Product1_dotp_1/1
  t/3 -> mul_Dot_Product1_dotp_2/1
  t1/1 -> mul_Dot_Product1_dotp_0/2
  t1/2 -> mul_Dot_Product1_dotp_1/2
  t1/3 -> mul_Dot_Product1_dotp_2/2
  mul_Dot_Product1_dotp_0/1 -> Dot_Product11/2
  mul_Dot_Product1_dotp_1/1 -> Dot_Product11/1
  Dot_Product11/1 -> Dot_Product12/2
  mul_Dot_Product1_dotp_2/1 -> Dot_Product12/1

== system gm_combinedTxRx_ExternalMode/Combined TX and RX/Receiver HDL/Frame Recover/Equalization and Demodulation/DFE/DFE/DotProd_linear_inst1 ==
  in1 : Inport  OutDataTypeStr=fixdt(1, 16, 14)  PortDimensions=[5]  SampleTime=1e-06
      settings: SignalType=complex
  in2 : Inport  Port=2  OutDataTypeStr=fixdt(1, 16, 14)  PortDimensions=[5]  SampleTime=1e-06
      settings: SignalType=complex
  Dot_Product : Math  Operator=conj  SaturateOnIntegerOverflow=on
  Dot_Product{1..4} (4 alike) : Sum  AccumDataTypeStr=fixdt(1, 16, 14)  OutDataTypeStr=fixdt(1, 16, 14)  SampleTime=1e-06  SaturateOnIntegerOverflow=on
  mul_Dot_Product_dotp_{0..4} (5 alike) : Product  Inputs=**  OutDataTypeStr=fixdt(1, 16, 14)  SampleTime=1e-06  SaturateOnIntegerOverflow=on
  t : Demux  Outputs=5
  t1 : Demux  Outputs=5
  out1 : Outport  OutDataTypeStr=fixdt(1, 16, 14)
      settings: SignalType=complex
  wires:
  in1/1 -> Dot_Product/1
  in2/1 -> t1/1
  Dot_Product4/1 -> out1/1
  Dot_Product/1 -> t/1
  t/1 -> mul_Dot_Product_dotp_0/1
  t/2 -> mul_Dot_Product_dotp_1/1
  t/3 -> mul_Dot_Product_dotp_2/1
  t/4 -> mul_Dot_Product_dotp_3/1
  t/5 -> mul_Dot_Product_dotp_4/1
  t1/1 -> mul_Dot_Product_dotp_0/2
  t1/2 -> mul_Dot_Product_dotp_1/2
  t1/3 -> mul_Dot_Product_dotp_2/2
  t1/4 -> mul_Dot_Product_dotp_3/2
  t1/5 -> mul_Dot_Product_dotp_4/2
  mul_Dot_Product_dotp_0/1 -> Dot_Product1/2
  mul_Dot_Product_dotp_1/1 -> Dot_Product1/1
  Dot_Product1/1 -> Dot_Product2/2
  mul_Dot_Product_dotp_2/1 -> Dot_Product2/1
  Dot_Product2/1 -> Dot_Product3/2
  mul_Dot_Product_dotp_3/1 -> Dot_Product3/1
  Dot_Product3/1 -> Dot_Product4/2
  mul_Dot_Product_dotp_4/1 -> Dot_Product4/1

== system gm_combinedTxRx_ExternalMode/Combined TX and RX/Receiver HDL/Frame Recover/Equalization and Demodulation/DFE/DFE/Forward Taps ==
  in0 : Inport  OutDataTypeStr=fixdt(1, 16, 14)  PortDimensions=[5]  SampleTime=1e-06
      settings: SignalType=complex
  Enable_out4 : EnablePort  OutDataTypeStr=boolean
  Forward Taps : UnitDelay  InitialCondition=[complex(0, 0) complex(0, 0) complex(1, 0) complex(0, 0) complex(0, 0)].'  SampleTime=1e-06
  out0 : Outport  OutDataTypeStr=fixdt(1, 16, 14)  PortDimensions=[5]  InitialOutput=0
      settings: SignalType=complex
  wires:
  Forward Taps/1 -> out0/1
  in0/1 -> Forward Taps/1

== system gm_combinedTxRx_ExternalMode/Combined TX and RX/Receiver HDL/Frame Recover/Equalization and Demodulation/DFE/DFE/InputBuffer_tap0 ==
  in0 : Inport  OutDataTypeStr=fixdt(1, 16, 14)  SampleTime=1e-06
      settings: SignalType=complex
  Enable_out4 : EnablePort  OutDataTypeStr=boolean
  InputBuffer_tap0 : Delay  DelayLength=hex2num('3ff0000000000000')  InputProcessing=Inherited
  out0 : Outport  OutDataTypeStr=fixdt(1, 16, 14)  InitialOutput=0
      settings: SignalType=complex
  wires:
  InputBuffer_tap0/1 -> out0/1
  in0/1 -> InputBuffer_tap0/1

== system gm_combinedTxRx_ExternalMode/Combined TX and RX/Receiver HDL/Frame Recover/Equalization and Demodulation/DFE/DFE/InputBuffer_tap1 ==
  in0 : Inport  OutDataTypeStr=fixdt(1, 16, 14)  SampleTime=1e-06
      settings: SignalType=complex
  Enable_out4 : EnablePort  OutDataTypeStr=boolean
  InputBuffer_tap1 : Delay  DelayLength=hex2num('3ff0000000000000')  InputProcessing=Inherited
  out0 : Outport  OutDataTypeStr=fixdt(1, 16, 14)  InitialOutput=0
      settings: SignalType=complex
  wires:
  InputBuffer_tap1/1 -> out0/1
  in0/1 -> InputBuffer_tap1/1

== system gm_combinedTxRx_ExternalMode/Combined TX and RX/Receiver HDL/Frame Recover/Equalization and Demodulation/DFE/DFE/InputBuffer_tap2 ==
  in0 : Inport  OutDataTypeStr=fixdt(1, 16, 14)  SampleTime=1e-06
      settings: SignalType=complex
  Enable_out4 : EnablePort  OutDataTypeStr=boolean
  InputBuffer_tap2 : Delay  DelayLength=hex2num('3ff0000000000000')  InputProcessing=Inherited
  out0 : Outport  OutDataTypeStr=fixdt(1, 16, 14)  InitialOutput=0
      settings: SignalType=complex
  wires:
  InputBuffer_tap2/1 -> out0/1
  in0/1 -> InputBuffer_tap2/1

== system gm_combinedTxRx_ExternalMode/Combined TX and RX/Receiver HDL/Frame Recover/Equalization and Demodulation/DFE/DFE/InputBuffer_tap3 ==
  in0 : Inport  OutDataTypeStr=fixdt(1, 16, 14)  SampleTime=1e-06
      settings: SignalType=complex
  Enable_out4 : EnablePort  OutDataTypeStr=boolean
  InputBuffer_tap3 : Delay  DelayLength=hex2num('3ff0000000000000')  InputProcessing=Inherited
  out0 : Outport  OutDataTypeStr=fixdt(1, 16, 14)  InitialOutput=0
      settings: SignalType=complex
  wires:
  InputBuffer_tap3/1 -> out0/1
  in0/1 -> InputBuffer_tap3/1

== system gm_combinedTxRx_ExternalMode/Combined TX and RX/Receiver HDL/Frame Recover/Equalization and Demodulation/DFE/DFE/InputBuffer_tap4 ==
  in0 : Inport  OutDataTypeStr=fixdt(1, 16, 14)  SampleTime=1e-06
      settings: SignalType=complex
  Enable_out4 : EnablePort  OutDataTypeStr=boolean
  InputBuffer_tap4 : Delay  DelayLength=hex2num('3ff0000000000000')  InputProcessing=Inherited
  out0 : Outport  OutDataTypeStr=fixdt(1, 16, 14)  InitialOutput=0
      settings: SignalType=complex
  wires:
  InputBuffer_tap4/1 -> out0/1
  in0/1 -> InputBuffer_tap4/1

== system gm_combinedTxRx_ExternalMode/Combined TX and RX/Receiver HDL/Frame Recover/Equalization and Demodulation/DFE/DFE/Map Symbol ==
  In1 : Inport  OutDataTypeStr=fixdt(1,16,14)  SampleTime=1e-06
  training : Inport  Port=2  OutDataTypeStr=fixdt(1,16,15)  SampleTime=1e-06
  reset : Inport  Port=3  SampleTime=1e-06
  Enable_out4 : Inport  Port=4  OutDataTypeStr=boolean  SampleTime=1e-06
  Decision Directed : Subsystem
  Delay : Subsystem
      settings: MinAlgLoopOccurrences=on
  HDL Counter : Subsystem
      settings: MinAlgLoopOccurrences=on
  Switch : Switch  Criteria=u2 > Threshold  Threshold=hex2num('406f400000000000')  OutDataTypeStr=fixdt(1, 16, 15)  SampleTime=1e-06
  d : Outport  InitialOutput=0
  wires:
  In1/1 -> Decision Directed/1(eqOut)
  training/1 -> Delay/1(in0)
  reset/1 -> HDL Counter/1(in0)
  Decision Directed/1(decision) -> Switch/1
  Delay/1(out0) -> Switch/3
  HDL Counter/1(out0) -> Switch/2
  Switch/1 -> d/1
  Enable_out4/1 -> HDL Counter/Enable, Delay/Enable

== system gm_combinedTxRx_ExternalMode/Combined TX and RX/Receiver HDL/Frame Recover/Equalization and Demodulation/DFE/DFE/Pipeline Delay1 ==
  in0 : Inport  OutDataTypeStr=int16  SampleTime=1e-06
  Enable_out4 : EnablePort  OutDataTypeStr=boolean
  Pipeline Delay1 : Delay  DelayLength=hex2num('3ff0000000000000')  InitialCondition=0  InputProcessing=Inherited
  out0 : Outport  OutDataTypeStr=int16  InitialOutput=0
  wires:
  Pipeline Delay1/1 -> out0/1
  in0/1 -> Pipeline Delay1/1

== system gm_combinedTxRx_ExternalMode/Combined TX and RX/Receiver HDL/Frame Recover/Equalization and Demodulation/DFE/DFE/Pipeline Delay2 ==
  in0 : Inport  OutDataTypeStr=fixdt(0, 16, 22)  SampleTime=1e-06
  Enable_out4 : EnablePort  OutDataTypeStr=boolean
  Pipeline Delay2 : Delay  DelayLength=hex2num('3ff0000000000000')  InitialCondition=0  InputProcessing=Inherited
  out0 : Outport  OutDataTypeStr=fixdt(0, 16, 22)  InitialOutput=0
  wires:
  Pipeline Delay2/1 -> out0/1
  in0/1 -> Pipeline Delay2/1

== system gm_combinedTxRx_ExternalMode/Combined TX and RX/Receiver HDL/Frame Recover/Gardner Timing Recovery/Gardner TED Blocks/Imag Error/Delay ==
  in0 : Inport  OutDataTypeStr=fixdt(1, 16, 10)  SampleTime=1e-06
  Enable_out2 : EnablePort  OutDataTypeStr=boolean
  Delay : Delay  DelayLength=hex2num('3ff0000000000000')  InitialCondition=0  InputProcessing=Inherited
  out0 : Outport  OutDataTypeStr=fixdt(1, 16, 10)  InitialOutput=0
  wires:
  Delay/1 -> out0/1
  in0/1 -> Delay/1

== system gm_combinedTxRx_ExternalMode/Combined TX and RX/Receiver HDL/Frame Recover/Gardner Timing Recovery/Gardner TED Blocks/Imag Error/TED Buffer Update1 ==
  new data : Inport  SampleTime=1e-06
  strobe sum : Inport  Port=2  SampleTime=1e-06
  Enable_out2 : Inport  Port=3  OutDataTypeStr=boolean  SampleTime=1e-06
  Delay : Subsystem
      settings: MinAlgLoopOccurrences=on
  Delay1 : Subsystem
      settings: MinAlgLoopOccurrences=on
  Delay2 : Subsystem
      settings: MinAlgLoopOccurrences=on
  Delay3 : Subsystem
      settings: MinAlgLoopOccurrences=on
  Multiport Switch{,1..3} (4 alike) : MultiPortSwitch  DataPortOrder=Zero-based contiguous  DiagnosticForDefault=None  OutDataTypeStr=fixdt(1, 16, 10)  SampleTime=1e-06
  Zero bit : Constant  Value=fi(0,1,16,13,'hex','0000')  OutDataTypeStr=fixdt(1, 16, 13)  SampleTime=-1
  Middle Indx : Outport  InitialOutput=0
  oldest : Outport  Port=2  InitialOutput=0
  wires:
  new data/1 -> Multiport Switch3/4, Multiport Switch3/3
  strobe sum/1 -> Multiport Switch3/1, Multiport Switch2/1, Multiport Switch1/1, Multiport Switch/1
  Delay/1(out0) -> Multiport Switch/2
  Delay1/1(out0) -> Multiport Switch1/2, Multiport Switch/3
  Delay2/1(out0) -> Multiport Switch2/2, Multiport Switch1/3, Multiport Switch/4
  Delay3/1(out0) -> Multiport Switch3/2, Multiport Switch2/3, Multiport Switch1/4
  Multiport Switch/1 -> Delay/1(in0), oldest/1
  Multiport Switch1/1 -> Delay1/1(in0)
  Multiport Switch2/1 -> Delay2/1(in0), Middle Indx/1
  Multiport Switch3/1 -> Delay3/1(in0)
  Zero bit/1 -> Multiport Switch2/4
  Enable_out2/1 -> Delay3/Enable, Delay2/Enable, Delay1/Enable, Delay/Enable

== system gm_combinedTxRx_ExternalMode/Combined TX and RX/Receiver HDL/Frame Recover/Gardner Timing Recovery/Gardner TED Blocks/Real Error/Delay ==
  in0 : Inport  OutDataTypeStr=fixdt(1, 16, 10)  SampleTime=1e-06
  Enable_out2 : EnablePort  OutDataTypeStr=boolean
  Delay : Delay  DelayLength=hex2num('3ff0000000000000')  InitialCondition=0  InputProcessing=Inherited
  out0 : Outport  OutDataTypeStr=fixdt(1, 16, 10)  InitialOutput=0
  wires:
  Delay/1 -> out0/1
  in0/1 -> Delay/1
